simulink model "ex_model_Top"  (R2022b)
settings: Solver=FixedStepAuto  StartTime=0.0  StopTime=10.0  RelTol=1e-3
settings Model: Creator=amyyang  LastModifiedBy=amyyang
settings OptimizationCC: DefaultParameterBehavior=Inlined  EnhancedBackFolding=on  PassReuseOutputArgsAs=Individual arguments  ZeroExternalMemoryAtStartup=off  ZeroInternalMemoryAtStartup=off  OptimizeBlockOrder=speed  DifferentSizesBufferReuse=on  OptimizationCustomize=off  EfficientTunableParamExpr=on
settings DebuggingCC: ParameterTunabilityLossMsg=error
settings ModelReferenceCC: ModelReferenceNumInstancesAllowed=Single
settings SFSimCC: MATLABDynamicMemAlloc=off
settings RTWCC: Description=Embedded Coder  SystemTargetFile=ert.tlc  TemplateMakefile=ert_default_tmf  Toolchain=LCC-win64 v2.4.1 | gmake (64-bit Windows)
settings CodeAppCC: ForceParamTrailComments=on  IgnoreCustomStorageClasses=off  MaxIdLength=256  OperatorAnnotations=on  SimulinkDataObjDesc=on  SFDataObjDesc=on  InsertBlockDesc=on
settings ERTTargetCC: TargetLangStandard=C99 (ISO)  GenerateSampleERTMain=on  InlinedParameterPlacement=NonHierarchical  ERTCustomFileTemplate=example_file_process.tlc

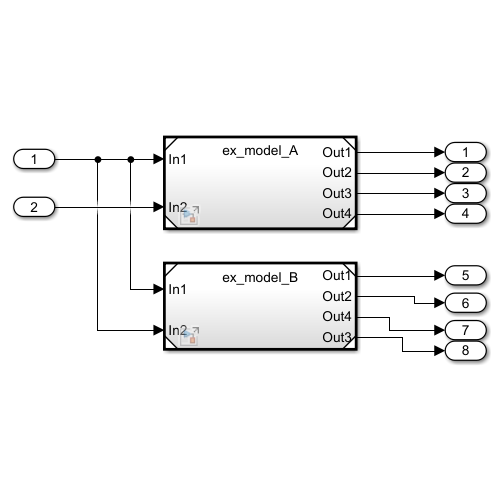
[thumbnail: Simulink's stored preview of the top-level diagram]
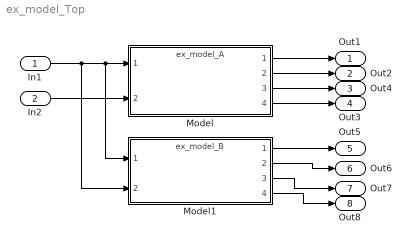
== system ex_model_Top ==
  In1 : Inport
  In2 : Inport  Port=2
  Model : ModelReference  ModelNameDialog=ex_model_A.slx  SimulationMode=Normal  ModelReferenceVersion=1.27
  Model1 : ModelReference  ModelNameDialog=ex_model_B.slx  SimulationMode=Normal  ModelReferenceVersion=1.31
  Out1 : Outport
  Out2 : Outport  Port=2
  Out4 : Outport  Port=3
  Out3 : Outport  Port=4
  Out5 : Outport  Port=5
  Out6 : Outport  Port=6
  Out7 : Outport  Port=7
  Out8 : Outport  Port=8
  wires:
  In1/1 -> Model/1, Model1/1, Model1/2
  In2/1 -> Model/2
  Model/1 -> Out1/1
  Model/2 -> Out2/1
  Model/3 -> Out4/1
  Model/4 -> Out3/1
  Model1/2 -> Out6/1
  Model1/1 -> Out5/1
  Model1/3 -> Out7/1
  Model1/4 -> Out8/1
